simulink model "dynamic_vibra"  (R2020a)
settings: Solver=VariableStepAuto  StartTime=0.0  StopTime=10.0  RelTol=1e-3
model workspace (MAT data in the model file):
  b = 50
  k1 = 50
  k12 = 15
  m1 = 100
  m2 = 4
settings Model: Creator=Shubham  LastModifiedBy=Shubham

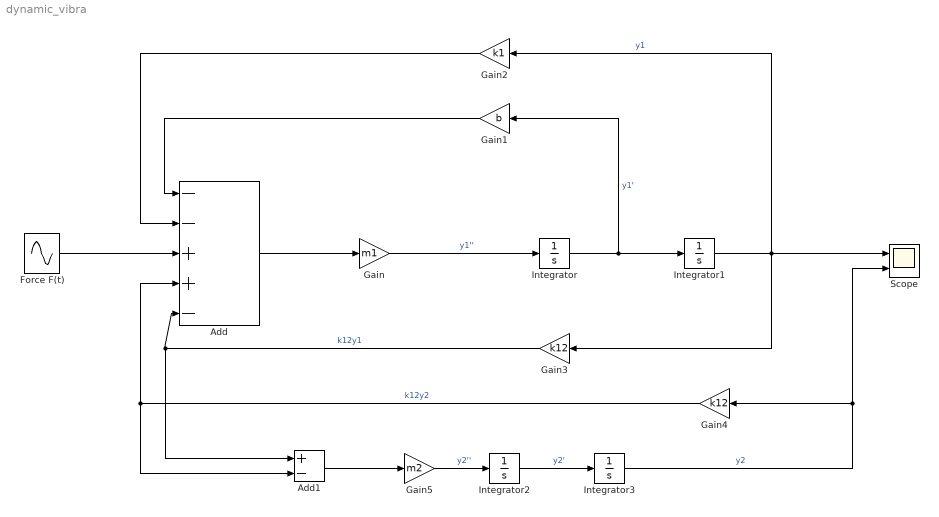
== system dynamic_vibra ==
  Add : Sum  Inputs=--++-
  Add1 : Sum  Inputs=+-
  Force F(t) : Sin  SampleTime=0
  Gain : Gain  Gain=m1
  Gain1 : Gain  Gain=b
  Gain2 : Gain  Gain=k1
  Gain3 : Gain  Gain=k12
  Gain4 : Gain  Gain=k12
  Gain5 : Gain  Gain=m2
  Integrator{,1..3} (4 alike) : Integrator
  Scope : Scope  NumInputPorts=2
  wires:
  Gain2/1 -> Add/2
  Integrator/1 -> Gain1/1, Integrator1/1  "y1'"
  Gain1/1 -> Add/1
  Gain/1 -> Integrator/1  "y1''"
  Gain4/1 -> Add1/2, Add/4  "k12y2"
  Gain3/1 -> Add1/1, Add/5  "k12y1"
  Force F(t)/1 -> Add/3
  Gain5/1 -> Integrator2/1  "y2''"
  Integrator1/1 -> Gain3/1, Gain2/1, Scope/1  "y1"
  Integrator2/1 -> Integrator3/1  "y2'"
  Integrator3/1 -> Gain4/1, Scope/2  "y2"
  Add/1 -> Gain/1
  Add1/1 -> Gain5/1
